simulink model "sm_stewart_platform"  (R2021b)
settings: Solver=ode45  StartTime=0.0  StopTime=40  MaxStep=0.2  RelTol=1e-3  EnableMultiTasking=on
model workspace (MAT data in the model file):
  g_density = 5
values from neighbouring files (symbols this model uses):
  B = zeros(3, 6)    [sm_stewart_platform_setup.m]
  nom_length = params.lower_leg_length + params.upper_leg_length +      2 * params.flange_length    [sm_stewart_platform_setup.m]
  P = rotation3(-pi/3, [0 0 1]) * P    [sm_stewart_platform_setup.m]
  s = cos(angle / 2)    [sm_stewart_platform_setup.m]
undefined symbols (not defined in the file or in its folder): X, Y, Z
libraries: sm_lib x20, sm_stewart_platform_lib x8, nesl_utility x4
(part 3 of 3)

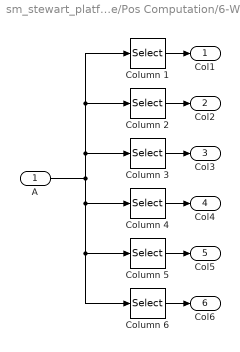
== system sm_stewart_platform/Stewart Platform System/Inverse Kinematics Module/Pos Computation/6-Way Column Splitter ==
  A : Inport
  Column 1 : Selector  NumberOfDimensions=2  InputPortWidth=3  IndexOptions=Select all,Index vector (dialog)  Indices=-1,1  OutputSizes=1
  Column 2 : Selector  NumberOfDimensions=2  InputPortWidth=3  IndexOptions=Select all,Index vector (dialog)  Indices=-1,2  OutputSizes=1
  Column 3 : Selector  NumberOfDimensions=2  InputPortWidth=3  IndexOptions=Select all,Index vector (dialog)  Indices=-1,3  OutputSizes=1
  Column 4 : Selector  NumberOfDimensions=2  InputPortWidth=3  IndexOptions=Select all,Index vector (dialog)  Indices=-1,4  OutputSizes=1
  Column 5 : Selector  NumberOfDimensions=2  InputPortWidth=3  IndexOptions=Select all,Index vector (dialog)  Indices=-1,5  OutputSizes=1
  Column 6 : Selector  NumberOfDimensions=2  InputPortWidth=3  IndexOptions=Select all,Index vector (dialog)  Indices=-1,6  OutputSizes=1
  Col1 : Outport  VectorParamsAs1DForOutWhenUnconnected=off
  Col2 : Outport  Port=2  VectorParamsAs1DForOutWhenUnconnected=off
  Col3 : Outport  Port=3  VectorParamsAs1DForOutWhenUnconnected=off
  Col4 : Outport  Port=4  VectorParamsAs1DForOutWhenUnconnected=off
  Col5 : Outport  Port=5  VectorParamsAs1DForOutWhenUnconnected=off
  Col6 : Outport  Port=6  VectorParamsAs1DForOutWhenUnconnected=off
  wires:
  A/1 -> Column 3/1, Column 2/1, Column 1/1, Column 4/1, Column 5/1, Column 6/1
  Column 1/1 -> Col1/1
  Column 2/1 -> Col2/1
  Column 3/1 -> Col3/1
  Column 4/1 -> Col4/1
  Column 5/1 -> Col5/1
  Column 6/1 -> Col6/1

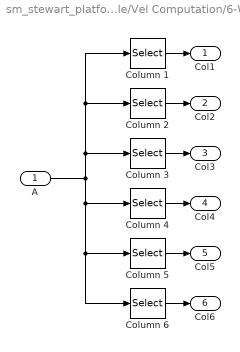
== system sm_stewart_platform/Stewart Platform System/Inverse Kinematics Module/Vel Computation/6-Way Column Splitter ==
  A : Inport
  Column 1 : Selector  NumberOfDimensions=2  InputPortWidth=3  IndexOptions=Select all,Index vector (dialog)  Indices=-1,1  OutputSizes=1
  Column 2 : Selector  NumberOfDimensions=2  InputPortWidth=3  IndexOptions=Select all,Index vector (dialog)  Indices=-1,2  OutputSizes=1
  Column 3 : Selector  NumberOfDimensions=2  InputPortWidth=3  IndexOptions=Select all,Index vector (dialog)  Indices=-1,3  OutputSizes=1
  Column 4 : Selector  NumberOfDimensions=2  InputPortWidth=3  IndexOptions=Select all,Index vector (dialog)  Indices=-1,4  OutputSizes=1
  Column 5 : Selector  NumberOfDimensions=2  InputPortWidth=3  IndexOptions=Select all,Index vector (dialog)  Indices=-1,5  OutputSizes=1
  Column 6 : Selector  NumberOfDimensions=2  InputPortWidth=3  IndexOptions=Select all,Index vector (dialog)  Indices=-1,6  OutputSizes=1
  Col1 : Outport  VectorParamsAs1DForOutWhenUnconnected=off
  Col2 : Outport  Port=2  VectorParamsAs1DForOutWhenUnconnected=off
  Col3 : Outport  Port=3  VectorParamsAs1DForOutWhenUnconnected=off
  Col4 : Outport  Port=4  VectorParamsAs1DForOutWhenUnconnected=off
  Col5 : Outport  Port=5  VectorParamsAs1DForOutWhenUnconnected=off
  Col6 : Outport  Port=6  VectorParamsAs1DForOutWhenUnconnected=off
  wires:
  A/1 -> Column 3/1, Column 2/1, Column 1/1, Column 4/1, Column 5/1, Column 6/1
  Column 1/1 -> Col1/1
  Column 2/1 -> Col2/1
  Column 3/1 -> Col3/1
  Column 4/1 -> Col4/1
  Column 5/1 -> Col5/1
  Column 6/1 -> Col6/1

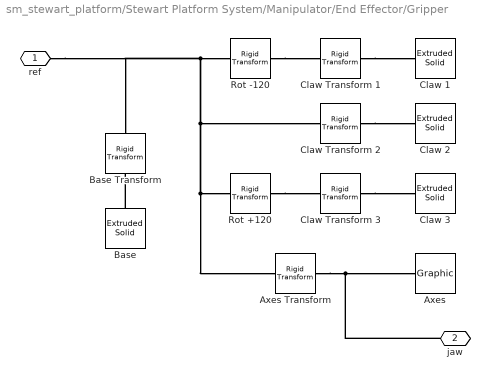
== system sm_stewart_platform/Stewart Platform System/Manipulator/End Effector/Gripper ==
  Axes : sm_lib/Body Elements/Graphic  GraphicType=Marker  MarkerShape=Frame  MarkerSize=25  MarkerSizeUnits=m  GraphicVisPropType=SimpleVisualProperties  GraphicDiffuseColor=[0.0 0.0 0.0]  GraphicSpecularColor=[0.2 0.2 0.2]  GraphicAmbientColor=[0.5 0.5 0.5]  GraphicEmissiveColor=[0.0 0.0 0.0 1.0]  GraphicShininess=24.0  GraphicOpacity=1.0
  Axes Transform : sm_lib/Frames and Transforms/Rigid Transform  TranslationMethod=StandardAxis  TranslationStandardOffset=claw_length  TranslationLengthUnit=cm  TranslationStandardAxis=+Z  TranslationCartesianOffset=[0 0 0]  TranslationROffset=0  TranslationROffsetUnits=m  TranslationZOffset=0  TranslationZOffsetUnits=m  TranslationThetaOffset=0  TranslationThetaOffsetUnits=deg  RotationMethod=None  RotationAngleUnits=deg  RotationStandardAxis=+Z  RotationAngle=0  RotationArbitraryAxis=[0 0 1]  FollAlignAxisA=+X  BaseAlignAxisA=+Y  FollAlignAxisB=+Y  BaseAlignAxisB=+Z  RotationSequenceAxes=FollowerAxes  RotationSequence=XYX  RotationSequenceAngles=[0 0 0]  RotationSequenceAnglesUnits=deg  RotationMatrix=[1 0 0; 0 1 0; 0 0 1]
  Base : sm_lib/Body Elements/Extruded Solid  GraphicAmbientColor=[0.1 0.1 0]  BasedOnType=Density  CenterOfMass=[0 0 0]  CenterOfMassUnits=m  GraphicDiffuseColor=[0.9 0.75 0] * 0.8  ExportConvexHullGeometry=off  ExtrusionCrossSection=[p1 p2 p3 p4 p5 p6]'  ExtrusionCrossSectionUnits=cm  Density=g_density  DensityUnits=g/cm^3  DoExposeReferenceFrame=on  GraphicEmissiveColor=[0.0 0.0 0.0]  ExportEntireGeometry=off  ExtrusionLength=base_thick  ExtrusionLengthUnits=cm  ExtrusionType=General  SerializedFrames=<Frames/>  MarkerShape=Sphere  MarkerSize=1  GraphicType=FromGeometry  InertiaType=CalculateFromGeometry  Mass=1  MassUnits=kg  MomentsOfInertia=[1 1 1]  MomentsOfInertiaUnits=kg*m^2  PolygonNumSides=1  GraphicOpacity=1  PolygonOuterRadius=1  PolygonOuterRadiusUnits=m  ProductsOfInertia=[0 0 0]  ProductsOfInertiaUnits=kg*m^2  GraphicShininess=80  GraphicSpecularColor=[0.9 0.75 0] * 0.8  GraphicVisPropType=AdvancedVisualProperties
  Base Transform : sm_lib/Frames and Transforms/Rigid Transform  TranslationMethod=StandardAxis  TranslationStandardOffset=base_thick / 2  TranslationLengthUnit=cm  TranslationStandardAxis=-Z  TranslationCartesianOffset=[0 0 0]  TranslationROffset=0  TranslationROffsetUnits=m  TranslationZOffset=0  TranslationZOffsetUnits=m  TranslationThetaOffset=0  TranslationThetaOffsetUnits=deg  RotationMethod=None  RotationAngleUnits=deg  RotationStandardAxis=+Z  RotationAngle=0  RotationArbitraryAxis=[0 0 1]  FollAlignAxisA=+X  BaseAlignAxisA=+Y  FollAlignAxisB=+Y  BaseAlignAxisB=+Z  RotationSequenceAxes=FollowerAxes  RotationSequence=XYX  RotationSequenceAngles=[0 0 0]  RotationSequenceAnglesUnits=deg  RotationMatrix=[1 0 0; 0 1 0; 0 0 1]
  Claw 1 : sm_lib/Body Elements/Extruded Solid  GraphicAmbientColor=[0.3 0.3 0]  BasedOnType=Density  CenterOfMass=[0 0 0]  CenterOfMassUnits=m  GraphicDiffuseColor=[0.9 0.75 0]  ExportConvexHullGeometry=off  ExtrusionCrossSection=[0 0; claw_width 0; claw_width/3 claw_length; 0 claw_length]  ExtrusionCrossSectionUnits=cm  Density=g_density  DensityUnits=g/cm^3  DoExposeReferenceFrame=on  GraphicEmissiveColor=[0.0 0.0 0.0]  ExportEntireGeometry=off  ExtrusionLength=claw_thick  ExtrusionLengthUnits=cm  ExtrusionType=General  SerializedFrames=<Frames/>  MarkerShape=Sphere  MarkerSize=1  GraphicType=FromGeometry  InertiaType=CalculateFromGeometry  Mass=1  MassUnits=kg  MomentsOfInertia=[1 1 1]  MomentsOfInertiaUnits=kg*m^2  PolygonNumSides=1  GraphicOpacity=1  PolygonOuterRadius=1  PolygonOuterRadiusUnits=m  ProductsOfInertia=[0 0 0]  ProductsOfInertiaUnits=kg*m^2  GraphicShininess=120  GraphicSpecularColor=[0.9 0.75 0]  GraphicVisPropType=AdvancedVisualProperties
  Claw 2 : sm_lib/Body Elements/Extruded Solid  GraphicAmbientColor=[0.3 0.3 0]  BasedOnType=Density  CenterOfMass=[0 0 0]  CenterOfMassUnits=m  GraphicDiffuseColor=[0.9 0.75 0]  ExportConvexHullGeometry=off  ExtrusionCrossSection=[0 0; claw_width 0; claw_width/3 claw_length; 0 claw_length]  ExtrusionCrossSectionUnits=cm  Density=g_density  DensityUnits=g/cm^3  DoExposeReferenceFrame=on  GraphicEmissiveColor=[0.0 0.0 0.0]  ExportEntireGeometry=off  ExtrusionLength=claw_thick  ExtrusionLengthUnits=cm  ExtrusionType=General  SerializedFrames=<Frames/>  MarkerShape=Sphere  MarkerSize=1  GraphicType=FromGeometry  InertiaType=CalculateFromGeometry  Mass=1  MassUnits=kg  MomentsOfInertia=[1 1 1]  MomentsOfInertiaUnits=kg*m^2  PolygonNumSides=1  GraphicOpacity=1  PolygonOuterRadius=1  PolygonOuterRadiusUnits=m  ProductsOfInertia=[0 0 0]  ProductsOfInertiaUnits=kg*m^2  GraphicShininess=120  GraphicSpecularColor=[0.9 0.75 0]  GraphicVisPropType=AdvancedVisualProperties
  Claw 3 : sm_lib/Body Elements/Extruded Solid  GraphicAmbientColor=[0.3 0.3 0]  BasedOnType=Density  CenterOfMass=[0 0 0]  CenterOfMassUnits=m  GraphicDiffuseColor=[0.9 0.75 0]  ExportConvexHullGeometry=off  ExtrusionCrossSection=[0 0; claw_width 0; claw_width/3 claw_length; 0 claw_length]  ExtrusionCrossSectionUnits=cm  Density=g_density  DensityUnits=g/cm^3  DoExposeReferenceFrame=on  GraphicEmissiveColor=[0.0 0.0 0.0]  ExportEntireGeometry=off  ExtrusionLength=claw_thick  ExtrusionLengthUnits=cm  ExtrusionType=General  SerializedFrames=<Frames/>  MarkerShape=Sphere  MarkerSize=1  GraphicType=FromGeometry  InertiaType=CalculateFromGeometry  Mass=1  MassUnits=kg  MomentsOfInertia=[1 1 1]  MomentsOfInertiaUnits=kg*m^2  PolygonNumSides=1  GraphicOpacity=1  PolygonOuterRadius=1  PolygonOuterRadiusUnits=m  ProductsOfInertia=[0 0 0]  ProductsOfInertiaUnits=kg*m^2  GraphicShininess=120  GraphicSpecularColor=[0.9 0.75 0]  GraphicVisPropType=AdvancedVisualProperties
  Claw Transform 1 : sm_lib/Frames and Transforms/Rigid Transform  TranslationMethod=StandardAxis  TranslationStandardOffset=claw_width  TranslationLengthUnit=cm  TranslationStandardAxis=+Y  TranslationCartesianOffset=[0 0 0]  TranslationROffset=0  TranslationROffsetUnits=m  TranslationZOffset=0  TranslationZOffsetUnits=m  TranslationThetaOffset=0  TranslationThetaOffsetUnits=deg  RotationMethod=AlignedAxes  RotationAngleUnits=deg  RotationStandardAxis=+Z  RotationAngle=0  RotationArbitraryAxis=[0 0 1]  FollAlignAxisA=+X  BaseAlignAxisA=+Y  FollAlignAxisB=+Y  BaseAlignAxisB=+Z  RotationSequenceAxes=FollowerAxes  RotationSequence=XYX  RotationSequenceAngles=[0 0 0]  RotationSequenceAnglesUnits=deg  RotationMatrix=[1 0 0; 0 1 0; 0 0 1]
  Claw Transform 2 : sm_lib/Frames and Transforms/Rigid Transform  TranslationMethod=StandardAxis  TranslationStandardOffset=claw_width  TranslationLengthUnit=cm  TranslationStandardAxis=+Y  TranslationCartesianOffset=[0 0 0]  TranslationROffset=0  TranslationROffsetUnits=m  TranslationZOffset=0  TranslationZOffsetUnits=m  TranslationThetaOffset=0  TranslationThetaOffsetUnits=deg  RotationMethod=AlignedAxes  RotationAngleUnits=deg  RotationStandardAxis=+Z  RotationAngle=0  RotationArbitraryAxis=[0 0 1]  FollAlignAxisA=+X  BaseAlignAxisA=+Y  FollAlignAxisB=+Y  BaseAlignAxisB=+Z  RotationSequenceAxes=FollowerAxes  RotationSequence=XYX  RotationSequenceAngles=[0 0 0]  RotationSequenceAnglesUnits=deg  RotationMatrix=[1 0 0; 0 1 0; 0 0 1]
  Claw Transform 3 : sm_lib/Frames and Transforms/Rigid Transform  TranslationMethod=StandardAxis  TranslationStandardOffset=claw_width  TranslationLengthUnit=cm  TranslationStandardAxis=+Y  TranslationCartesianOffset=[0 0 0]  TranslationROffset=0  TranslationROffsetUnits=m  TranslationZOffset=0  TranslationZOffsetUnits=m  TranslationThetaOffset=0  TranslationThetaOffsetUnits=deg  RotationMethod=AlignedAxes  RotationAngleUnits=deg  RotationStandardAxis=+Z  RotationAngle=0  RotationArbitraryAxis=[0 0 1]  FollAlignAxisA=+X  BaseAlignAxisA=+Y  FollAlignAxisB=+Y  BaseAlignAxisB=+Z  RotationSequenceAxes=FollowerAxes  RotationSequence=XYX  RotationSequenceAngles=[0 0 0]  RotationSequenceAnglesUnits=deg  RotationMatrix=[1 0 0; 0 1 0; 0 0 1]
  Rot +120 : sm_lib/Frames and Transforms/Rigid Transform  TranslationMethod=None  TranslationStandardOffset=0  TranslationLengthUnit=m  TranslationStandardAxis=+Z  TranslationCartesianOffset=[0 0 0]  TranslationROffset=0  TranslationROffsetUnits=m  TranslationZOffset=0  TranslationZOffsetUnits=m  TranslationThetaOffset=0  TranslationThetaOffsetUnits=deg  RotationMethod=StandardAxis  RotationAngleUnits=deg  RotationStandardAxis=+Z  RotationAngle=+120  RotationArbitraryAxis=[0 0 1]  FollAlignAxisA=+X  BaseAlignAxisA=+Y  FollAlignAxisB=+Y  BaseAlignAxisB=+Z  RotationSequenceAxes=FollowerAxes  RotationSequence=XYX  RotationSequenceAngles=[0 0 0]  RotationSequenceAnglesUnits=deg  RotationMatrix=[1 0 0; 0 1 0; 0 0 1]
  Rot -120 : sm_lib/Frames and Transforms/Rigid Transform  TranslationMethod=None  TranslationStandardOffset=0  TranslationLengthUnit=m  TranslationStandardAxis=+Z  TranslationCartesianOffset=[0 0 0]  TranslationROffset=0  TranslationROffsetUnits=m  TranslationZOffset=0  TranslationZOffsetUnits=m  TranslationThetaOffset=0  TranslationThetaOffsetUnits=deg  RotationMethod=StandardAxis  RotationAngleUnits=deg  RotationStandardAxis=+Z  RotationAngle=-120  RotationArbitraryAxis=[0 0 1]  FollAlignAxisA=+X  BaseAlignAxisA=+Y  FollAlignAxisB=+Y  BaseAlignAxisB=+Z  RotationSequenceAxes=FollowerAxes  RotationSequence=XYX  RotationSequenceAngles=[0 0 0]  RotationSequenceAnglesUnits=deg  RotationMatrix=[1 0 0; 0 1 0; 0 0 1]
  ref : PMIOPort  Side=Left
  jaw : PMIOPort  Port=2  Side=Right
  connections:
  Claw Transform 1/RConn1 -- Claw 1/RConn1
  Claw Transform 2/LConn1 -- ref/RConn1 -- Base Transform/LConn1 -- Rot -120/LConn1 -- Axes Transform/LConn1 -- Rot +120/LConn1
  Claw Transform 2/RConn1 -- Claw 2/RConn1
  Claw Transform 3/RConn1 -- Claw 3/RConn1
  Base/RConn1 -- Base Transform/RConn1
  Axes Transform/RConn1 -- Axes/RConn1 -- jaw/RConn1
  Rot -120/RConn1 -- Claw Transform 1/LConn1
  Rot +120/RConn1 -- Claw Transform 3/LConn1
